simulink model "fpdun"  (R2016a)
settings: Solver=VariableStepAuto  StartTime=0.0  StopTime=10.0  RelTol=1e-3
settings Model: Creator=Memoir  LastModifiedBy=Memoir

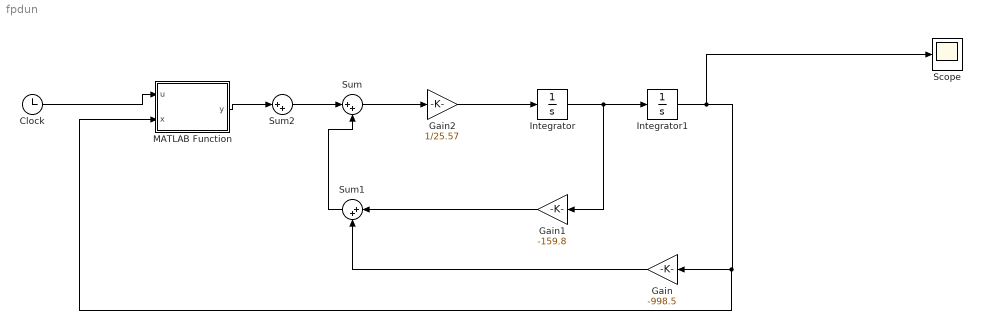
== system fpdun ==
  Clock : Clock
  Gain : Gain  Gain=-998.5
  Gain1 : Gain  Gain=-159.8
  Gain2 : Gain  Gain=1/25.57
  Integrator : Integrator
  Integrator1 : Integrator
  MATLAB Function : MATLAB Function  TreatAsAtomicUnit=on
  Scope : Scope
  Sum : Sum  Inputs=|++
  Sum1 : Sum  Inputs=|++
  Sum2 : Sum  Inputs=|++
  wires:
  Integrator/1 -> Gain1/1, Integrator1/1
  Integrator1/1 -> Scope/1, MATLAB Function/2(x), Gain/1
  Sum/1 -> Gain2/1
  Gain2/1 -> Integrator/1
  Gain/1 -> Sum1/2
  Gain1/1 -> Sum1/1
  Sum1/1 -> Sum/2
  Clock/1 -> MATLAB Function/1(u)
  MATLAB Function/1(y) -> Sum2/1
  Sum2/1 -> Sum/1

== matlab function fpdun/MATLAB Function ==
  data: u input size=1; y output size=1; x input
function y = fcn(u,x)
%#codegen
%参数计算
h = 2; %水深
T = 1.5; % 周期
H = 0.15; % 波高
Cv = 1.08; % 绕射系数
R = 0.18; %浮子半径
rho = 1000; %水密度
g = 9.8; %重力加速度
coder.extrinsic('myFunc')
coder.extrinsic('myFunc1')
L = 0;
L = myFunc(h,T) % 波长
k_ = 2*pi/L; % 波数
w = 2*pi/T; % 波浪频率
temp = 0;
temp = myFunc1(k_,R);
d=0.25-x+H/2*cos(k_*x-2*pi*u/T);%浮子吃水 
%结果
y = 1; %定义y类型
y = Cv*rho*g*pi*H*R*cosh(k_*(h-d))*temp*cos(w*u)/(k_*cosh(k_*h));
